simulink library "tqd"  (R2021b)
settings: Solver=VariableStepAuto  StartTime=0.0  StopTime=10.0  RelTol=1e-3
undefined symbols (not defined in the file or in its folder): ATQD_APSDecReq_X_kph, ATQD_APSDecReq_Y_mps2, ATQD_APSDecReqCMD_X_kph, ATQD_APSDecReqTs_X_pct, ATQD_APSDecTimeGain_X_Deg, ATQD_APSDecTimeGain_Y_s, ATQD_APSReqLowSpd_X_Deg, ATQD_AutoHoldReleaseBPS_X_Deg, ATQD_AWDLoadTrqnsGain_X_kg, ATQD_AWDLoadTrqnsGain_Y_pct, ATQD_BOSEnBPSPosn_X_kph, ATQD_BOSMap_X_rpm, ATQD_BOSMap_Y_pct, ATQD_CreepBaseTqD_X_kph, ATQD_CreepBaseTqD_Y_Deg, ATQD_CreepBaseTqR_X_kph, ATQD_CreepBaseTqR_Y_Deg, ATQD_CreepBPSDisPosn_X_Deg, ATQD_CreepBPSDisPosnR_X_Deg, ATQD_CreepBPSEnPosn_X_Deg, ATQD_CreepBPSEnPosnR_X_Deg, ATQD_CreepDeltaTq_X_kph, ATQD_CreepIterm_X_kph, ATQD_CreepIterm_Y_kph, ATQD_CreepItermMaxLimit_X_pct, ATQD_CreepPreloadTime_X_kph, ATQD_CreepPreloadTq_X_kph, ATQD_CreepPreloadTq_Y_s, ATQD_CreepProtTq_X_Deg, ATQD_CreepPterm_X_kph, ATQD_CreepPterm_Y_kph, ATQD_ECOTqMapD_X_rpm, ATQD_ECOTqMapD_Y_pct, ATQD_EOPDTqMapDCon_X_rpm, ATQD_EOPDTqMapDCon_Y_Deg, ATQD_EstInitVehWeight_X_c, ATQD_LHMRollGenMapD_X_rpm, ATQD_LHMRollGenMapD_Y_rpm, ATQD_LHMTqMapD_X_rpm, ATQD_LHMTqMapD_Y_pct, ATQD_NL1TqMapD_X_rpm, ATQD_NL1TqMapD_Y_pct, ATQD_NOPDTqMapDCon_X_rpm, ATQD_NOPDTqMapDCon_Y_Deg, ATQD_NRMRrEDUSpRat_X_rpm, ATQD_NRMRrEDUSpRat_Y_Nm, ATQD_OPDHoldDownRelDelay_X_Deg, ATQD_OPDHoldEnSpd_X_Deg, ATQD_OPDHoldRelDetTime_X_Deg, ATQD_OPDHoldReleaseTq_X_Deg, ATQD_OrigPedTqLowLim_X_Deg, ATQD_OrigPedTqLowLim_Y_pct, ATQD_PedalMapClimbUpLim_X_rpm, ATQD_PedalMapClimbUpLim_Y_Deg, ATQD_PreLoadTq_X_s, ATQD_RollGenMapEL1_X_rpm, ATQD_RollGenMapEL1_Y_rpm, ATQD_SL1TqMapD_X_rpm, ATQD_SL1TqMapD_Y_pct, ATQD_SlideRegenTqGain_X_Gps ... (+491)
libraries: hcu_lib x83, simulink x73, tqr x1
(part 19 of 19)

== stateflow chart tqd/TQD/TorqueDemand/Signal_convert/SWC2_Subsystem/Speed Setting Mode/MSA Speed Setting ON/MSASetSpd_241018 ==
  state MeterSpd
    state OFF_Error_Disable
      en:
      VTQD_MSASetSpd_raw32 =  min(VTQD_MSAActiveMetSpdHi_raw32, VTQD_SpdLim4SetSpd_raw32);
      VTQD_MSASetSpd_raw32 = max(VTQD_MSAActiveMetSpdLo_raw32, VTQD_MSASetSpd_raw32);
      VTQD_MSASavedSetSpd_raw32 = VTQD_MSASetSpd_raw32;
      du:
      VTQD_MSASetSpd_raw32 =  min(VTQD_MSAActiveMetSpdHi_raw32, VTQD_SpdLim4SetSpd_raw32);
      VTQD_MSASetSpd_raw32 = max(VTQD_MSAActiveMetSpdLo_raw32, VTQD_MSASetSpd_raw32);
      VTQD_MSASavedSetSpd_raw32 = VTQD_MSASetSpd_raw32;
    state Terminal
      %Do Nothing
    state Standby
      en:
      VTQD_MSASetSpd_raw32 =  min(VTQD_MSAActiveMetSpdHi_raw32, VTQD_SpdLim4SetSpd_raw32);
      VTQD_MSASetSpd_raw32 = max(VTQD_MSAActiveMetSpdLo_raw32, VTQD_MSASetSpd_raw32);
      VTQD_MSASavedSetSpd_raw32 = VTQD_MSASetSpd_raw32;
      du:
      VTQD_MSASetSpd_raw32 =  min(VTQD_MSAActiveMetSpdHi_raw32, VTQD_SpdLim4SetSpd_raw32);
      VTQD_MSASetSpd_raw32 = max(VTQD_MSAActiveMetSpdLo_raw32, VTQD_MSASetSpd_raw32);
      VTQD_MSASavedSetSpd_raw32 = VTQD_MSASetSpd_raw32;
    state Active_Override
      (default) -> (junction 749) : {VTQD_MSASetSpd_raw32 = VTQD_MSASavedSetSpd_raw32;}
      MeterSpd.Active_Override -> (junction 830) [order 1]
      (junction 830) -> (junction 834) [order 1] : [VTQD_DistanceUnit_flg == VINP_Distanceunit_flg || VTQD_MSASavedSetSpd_raw32 <= ONE_FLOAT]
      (junction 834) -> (junction 749) : {VTQD_MSASetSpd_raw32 = min(VTQD_MSAActiveMetSpdHi_raw32, VTQD_MSASavedSetSpd_raw32);
          |  VTQD_MSASavedSetSpd_raw32 = VTQD_MSASetSpd_raw32;}
      (junction 749) -> (junction 751) [order 1] : [VVMC_MSACrlSta_enum == ENUM_ADASMSASTA_ACTIVE]
      (junction 751) -> (junction 757) [order 1] : [VTQD_Set2MeterSpd_flg ||...
          |  VTQD_SetRoadSpdLim_flg]
      (junction 757) -> (junction 1111) [order 1] : [VTQD_Set2MeterSpd_flg]
      (junction 830) -> (junction 832) [order 2]
      (junction 837) -> (junction 834)
      (junction 749) -> (junction 798) [order 2]
      (junction 751) -> (junction 762) [order 2]
      (junction 757) -> (junction 759) [order 2] : {VTQD_MSASetSpd_raw32 =  min(VTQD_MSAActiveMetSpdHi_raw32, VTQD_SpdLim4SetSpd_raw32);
          |  VTQD_MSASetSpd_raw32 = max(VTQD_MSAActiveMetSpdLo_raw32, VTQD_MSASetSpd_raw32);
          |  VTQD_MSASavedSetSpd_raw32 = VTQD_MSASetSpd_raw32;
          |  VTQD_DistanceUnit_flg = VINP_Distanceunit_flg;}
      (junction 1111) -> (junction 1112) : {VTQD_MSASetSpd_raw32 =  min(VTQD_MSAActiveMetSpdHi_raw32, VVMC_MeterIndSpeed_raw32);
          |  VTQD_MSASetSpd_raw32 = max(VTQD_MSAActiveMetSpdLo_raw32, VTQD_MSASetSpd_raw32);
          |  VTQD_MSASavedSetSpd_raw32 = VTQD_MSASetSpd_raw32;
          |  VTQD_DistanceUnit_flg = VINP_Distanceunit_flg;}
      (junction 832) -> (junction 819) [order 1] : [VINP_Distanceunit_flg]
      (junction 832) -> (junction 833) [order 2] : {VTQD_MSASavedSetSpd_raw32 = (VTQD_MSASavedSetSpd_raw32 * MPH2KPH)}
      (junction 819) -> (junction 827) : {VTQD_MSASavedSetSpd_raw32 = (VTQD_MSASavedSetSpd_raw32 * KPH2MPH)}
      (junction 762) -> (junction 766) [order 1] : [(VTQD_SWC2ScrollUpSta_enum == ENUM_SWCBOTTONPRESS_SHORTPRESS ||...
          |   VTQD_SWC2ScrollDownSta_enum == ENUM_SWCBOTTONPRESS_SHORTPRESS)]
      (junction 766) -> (junction 771) [order 1] : [VTQD_SWC2ScrollUpSta_enum == ENUM_SWCBOTTONPRESS_SHORTPRESS]
      (junction 762) -> (junction 792) [order 2]
      (junction 766) -> (junction 779) [order 2] : {VTQD_MSASetSpd_raw32 =  min(VTQD_MSAActiveMetSpdHi_raw32, VTQD_MSASavedSetSpd_raw32 - ONE_FLOAT);
          |  VTQD_MSASetSpd_raw32 = max(VTQD_MSAActiveMetSpdLo_raw32, VTQD_MSASetSpd_raw32);
          |  VTQD_MSASavedSetSpd_raw32 = VTQD_MSASetSpd_raw32;
          |  VTQD_DistanceUnit_flg = VINP_Distanceunit_flg;}
      (junction 771) -> (junction 774) : {VTQD_MSASetSpd_raw32 =  min(VTQD_MSAActiveMetSpdHi_raw32, VTQD_MSASavedSetSpd_raw32 + ONE_FLOAT);
          |  VTQD_MSASetSpd_raw32 = max(VTQD_MSAActiveMetSpdLo_raw32, VTQD_MSASetSpd_raw32);
          |  VTQD_MSASavedSetSpd_raw32 = VTQD_MSASetSpd_raw32;
          |  VTQD_DistanceUnit_flg = VINP_Distanceunit_flg;}
      (junction 827) -> (junction 816) [order 1] : [VTQD_MSASavedSetSpd_raw32 < KTQD_MSAActiveMetSpdLoMPH_mph]
      (junction 833) -> (junction 817) [order 1] : [VTQD_MSASavedSetSpd_raw32 < KTQD_MSAActiveMetSpdLo_kph]
      (junction 816) -> (junction 820) : {VTQD_MSASavedSetSpd_raw32 = KTQD_MSAActiveMetSpdLoMPH_mph}
      (junction 833) -> (junction 828) [order 2]
      (junction 817) -> (junction 815) : {VTQD_MSASavedSetSpd_raw32 = KTQD_MSAActiveMetSpdLo_kph}
      (junction 827) -> (junction 818) [order 2]
      (junction 820) -> (junction 818)
      (junction 815) -> (junction 828)
      (junction 818) -> (junction 826)
      (junction 828) -> (junction 821)
      (junction 821) -> (junction 829) [order 1] : [VTQD_MSASavedSetSpd_raw32 > KTQD_MSAActiveMetSpdHi_kph]
      (junction 826) -> (junction 822) [order 1] : [VTQD_MSASavedSetSpd_raw32 > KTQD_MSAActiveMetSpdHiMPH_mph]
      (junction 821) -> (junction 823) [order 2]
      (junction 829) -> (junction 831) : {VTQD_MSASavedSetSpd_raw32 = KTQD_MSAActiveMetSpdHi_kph}
      (junction 826) -> (junction 835) [order 2]
      (junction 822) -> (junction 824) : {VTQD_MSASavedSetSpd_raw32 = KTQD_MSAActiveMetSpdHiMPH_mph}
      (junction 792) -> (junction 785) [order 1] : [(VTQD_SWC2ScrollUpSta_enum == ENUM_SWCBOTTONPRESS_LONGPRESS ||...
          |   VTQD_SWC2ScrollDownSta_enum == ENUM_SWCBOTTONPRESS_LONGPRESS)]
      (junction 785) -> (junction 790) [order 1] : [VTQD_SWC2ScrollUpSta_enum == ENUM_SWCBOTTONPRESS_LONGPRESS]
      (junction 831) -> (junction 823)
      (junction 824) -> (junction 835)
      (junction 785) -> (junction 793) [order 2] : {VTQD_MSASetSpd_raw32 = max(VTQD_MSAActiveMetSpdLo_raw32, ceil(VTQD_MSASavedSetSpd_raw32 / VTQD_SetSpdDeltaLong_raw32 - ONE_FLOAT) * VTQD_SetSpdDeltaLong_raw32);
          |  VTQD_MSASetSpd_raw32 = min (VTQD_MSAActiveMetSpdHi_raw32, VTQD_MSASetSpd_raw32);
          |  VTQD_MSASavedSetSpd_raw32 = VTQD_MSASetSpd_raw32;
          |  VTQD_DistanceUnit_flg = VINP_Distanceunit_flg;}
      (junction 792) -> (junction 809) [order 2] : {VTQD_MSASetSpd_raw32 = min(VTQD_MSAActiveMetSpdHi_raw32, ...
          |  VTQD_MSASavedSetSpd_raw32);
          |  VTQD_MSASetSpd_raw32 = max(VTQD_MSAActiveMetSpdLo_raw32, ...
          |  VTQD_MSASetSpd_raw32);
          |  VTQD_MSASavedSetSpd_raw32 = VTQD_MSASetSpd_raw32;
          |  VTQD_DistanceUnit_flg = VINP_Distanceunit_flg;}
          | %add20241113
      (junction 790) -> (junction 783) : {VTQD_MSASetSpd_raw32 = min(VTQD_MSAActiveMetSpdHi_raw32, floor(VTQD_MSASavedSetSpd_raw32 / VTQD_SetSpdDeltaLong_raw32 + ONE_FLOAT) * VTQD_SetSpdDeltaLong_raw32);
          |  VTQD_MSASetSpd_raw32 = max (VTQD_MSAActiveMetSpdLo_raw32, VTQD_MSASetSpd_raw32);
          |  VTQD_MSASavedSetSpd_raw32 = VTQD_MSASetSpd_raw32;
          |  VTQD_DistanceUnit_flg = VINP_Distanceunit_flg;}
      (junction 823) -> (junction 825)
      (junction 835) -> (junction 836)
      (junction 825) -> (junction 836)
      (junction 836) -> (junction 837)
      (junction 798) -> (junction 806) [order 1] : [VVMC_MSACrlSta_enum == ENUM_ADASMSASTA_UNLIMIT]
      (junction 806) -> (junction 804) [order 1] : [KTQD_ACCOVRDSpdAdj_flg &&...
          | (VTQD_Set2MeterSpd_flg ||...
          |  VTQD_SetRoadSpdLim_flg)]
      (junction 804) -> (junction 1115) [order 1] : [VTQD_Set2MeterSpd_flg]
      (junction 804) -> (junction 803) [order 2] : {VTQD_MSASetSpd_raw32 =  min(VTQD_MSAActiveMetSpdHi_raw32, VTQD_SpdLim4SetSpd_raw32);
          |  VTQD_MSASetSpd_raw32 = max(VTQD_MSAActiveMetSpdLo_raw32, VTQD_MSASetSpd_raw32);
          |  VTQD_MSASavedSetSpd_raw32 = VTQD_MSASetSpd_raw32;
          |  VTQD_DistanceUnit_flg = VINP_Distanceunit_flg;}
      (junction 1115) -> (junction 1116) : {VTQD_MSASetSpd_raw32 =  min(VTQD_MSAActiveMetSpdHi_raw32, VVMC_MeterIndSpeed_raw32);
          |  VTQD_MSASetSpd_raw32 = max(VTQD_MSAActiveMetSpdLo_raw32, VTQD_MSASetSpd_raw32);
          |  VTQD_MSASavedSetSpd_raw32 = VTQD_MSASetSpd_raw32;
          |  VTQD_DistanceUnit_flg = VINP_Distanceunit_flg;}
      (junction 798) -> (junction 807) [order 2] : {VTQD_MSASetSpd_raw32 = min(VTQD_MSAActiveMetSpdHi_raw32, ...
          |  VTQD_MSASavedSetSpd_raw32);
          |  VTQD_MSASetSpd_raw32 = max(VTQD_MSAActiveMetSpdLo_raw32, ...
          |  VTQD_MSASetSpd_raw32);
          |  VTQD_MSASavedSetSpd_raw32 = VTQD_MSASetSpd_raw32;
          |  VTQD_DistanceUnit_flg = VINP_Distanceunit_flg;}
          | %add20241113
      (junction 806) -> (junction 811) [order 2] : {VTQD_MSASetSpd_raw32 = min(VTQD_MSAActiveMetSpdHi_raw32, ...
          |  VTQD_MSASavedSetSpd_raw32);
          |  VTQD_MSASetSpd_raw32 = max(VTQD_MSAActiveMetSpdLo_raw32, ...
          |  VTQD_MSASetSpd_raw32);
          |  VTQD_MSASavedSetSpd_raw32 = VTQD_MSASetSpd_raw32;
          |  VTQD_DistanceUnit_flg = VINP_Distanceunit_flg;}
          | %add20241113
    (default) -> MeterSpd.OFF_Error_Disable [order 3]
    MeterSpd.Terminal -> MeterSpd.OFF_Error_Disable [order 2] : [VVMC_MSACrlSta_enum ~= ENUM_ADASMSASTA_ACTIVE &&...
        |  VVMC_MSACrlSta_enum ~= ENUM_ADASMSASTA_UNLIMIT]
    MeterSpd.OFF_Error_Disable -> MeterSpd.Terminal [order 2] : [VVMC_MSACrlSta_enum == ENUM_ADASMSASTA_ACTIVE ||...
        |  VVMC_MSACrlSta_enum == ENUM_ADASMSASTA_UNLIMIT]
    MeterSpd.Terminal -> MeterSpd.Active_Override [order 1] : [VVMC_MSACrlSta_enum == ENUM_ADASMSASTA_ACTIVE ||...
        |  VVMC_MSACrlSta_enum == ENUM_ADASMSASTA_UNLIMIT]
    MeterSpd.Active_Override -> MeterSpd.Terminal [order 2] : [VVMC_MSACrlSta_enum ~= ENUM_ADASMSASTA_ACTIVE &&...
        |  VVMC_MSACrlSta_enum ~= ENUM_ADASMSASTA_UNLIMIT]
    MeterSpd.OFF_Error_Disable -> MeterSpd.Standby [order 1] : [VVMC_MSACrlSta_enum == ENUM_ADASMSASTA_STANDBY]
    MeterSpd.Standby -> MeterSpd.OFF_Error_Disable [order 2] : [VVMC_MSACrlSta_enum ~= ENUM_ADASMSASTA_STANDBY]
    MeterSpd.Active_Override -> MeterSpd.Standby [order 1] : [VVMC_MSACrlSta_enum == ENUM_ADASMSASTA_STANDBY]
    MeterSpd.Standby -> MeterSpd.Active_Override [order 1] : [VVMC_MSACrlSta_enum == ENUM_ADASMSASTA_ACTIVE ||...
        |  VVMC_MSACrlSta_enum == ENUM_ADASMSASTA_UNLIMIT]
    (default) -> MeterSpd.Active_Override [order 2] : [VVMC_MSACrlSta_enum == ENUM_ADASMSASTA_ACTIVE ||...
        |  VVMC_MSACrlSta_enum == ENUM_ADASMSASTA_UNLIMIT]
    (default) -> MeterSpd.Standby [order 1] : [VVMC_MSACrlSta_enum == ENUM_ADASMSASTA_STANDBY]
  state RoadSpd
    state OFF_Error_Disable
      en:
      VTQD_MSASetSpd_raw32 =  min(VTQD_MSAActiveMetSpdHi_raw32, VTQD_SpdLim4SetSpd_raw32);
      VTQD_MSASetSpd_raw32 = max(VTQD_MSAActiveMetSpdLo_raw32, VTQD_MSASetSpd_raw32);
      VTQD_MSASavedSetSpd_raw32 = VTQD_MSASetSpd_raw32;
      du:
      VTQD_MSASetSpd_raw32 =  min(VTQD_MSAActiveMetSpdHi_raw32, VTQD_SpdLim4SetSpd_raw32);
      VTQD_MSASetSpd_raw32 = max(VTQD_MSAActiveMetSpdLo_raw32, VTQD_MSASetSpd_raw32);
      VTQD_MSASavedSetSpd_raw32 = VTQD_MSASetSpd_raw32;
    state Terminal
      %Do Nothing
    state Standby
      (default) -> (junction 987) : {VTQD_StandbyDisRoadSpd_flg = FALSE;}
      RoadSpd.Standby -> (junction 1029) [order 1]
      (junction 1029) -> (junction 1030) [order 1] : [VTQD_DistanceUnit_flg == VINP_Distanceunit_flg || VTQD_MSASavedSetSpd_raw32 <= ONE_FLOAT]
      (junction 1030) -> (junction 987) : {VTQD_MSASetSpd_raw32 = min(VTQD_MSAActiveMetSpdHi_raw32, VTQD_MSASavedSetSpd_raw32);
          |  VTQD_MSASavedSetSpd_raw32 = VTQD_MSASetSpd_raw32;}
      (junction 987) -> (junction 1102) [order 1] : [VTQD_RoadSpdActive2Standby_flg &&...
          | (VTQD_StandbyDisRoadSpd_flg || !VTQD_ADASSLIFSpdLimDet_flg)]
      (junction 1029) -> (junction 1031) [order 2]
      (junction 1048) -> (junction 1030)
      (junction 987) -> (junction 1104) [order 2]
      (junction 1102) -> (junction 999)
      (junction 1031) -> (junction 1032) [order 1] : [VINP_Distanceunit_flg]
      (junction 1031) -> (junction 1034) [order 2] : {VTQD_MSASavedSetSpd_raw32 = (VTQD_MSASavedSetSpd_raw32 * MPH2KPH)}
      (junction 1032) -> (junction 1028) : {VTQD_MSASavedSetSpd_raw32 = (VTQD_MSASavedSetSpd_raw32 * KPH2MPH)}
      (junction 1104) -> (junction 999) [order 1] : [VTQD_SWC2ScrollUpSta_enum ~= ENUM_SWCBOTTONPRESS_NOPRESS ||...
          |  VTQD_SWC2ScrollDownSta_enum ~= ENUM_SWCBOTTONPRESS_NOPRESS ||...
          |  VTQD_StandbyDisRoadSpd_flg]
      (junction 999) -> (junction 1000) [order 1] : [VTQD_SWC2ScrollUpSta_enum == ENUM_SWCBOTTONPRESS_SHORTPRESS ||...
          |  VTQD_SWC2ScrollDownSta_enum == ENUM_SWCBOTTONPRESS_SHORTPRESS]
      (junction 1000) -> (junction 1001) [order 1] : [VTQD_SWC2ScrollUpSta_enum == ENUM_SWCBOTTONPRESS_SHORTPRESS]
      (junction 1104) -> (junction 991) [order 2] : {VTQD_MSASetSpd_raw32 =  min(VTQD_MSAActiveMetSpdHi_raw32, VTQD_SpdLim4SetSpd_raw32);
          |  VTQD_MSASetSpd_raw32 = max(VTQD_MSAActiveMetSpdLo_raw32, VTQD_MSASetSpd_raw32);
          |  VTQD_MSASavedSetSpd_raw32 = VTQD_MSASetSpd_raw32;
          |  VTQD_DistanceUnit_flg = VINP_Distanceunit_flg;
          |  VTQD_RoadSpdActive2Standby_flg = FALSE;}
      (junction 999) -> (junction 1007) [order 2]
      (junction 1000) -> (junction 1005) [order 2] : {VTQD_MSASetSpd_raw32 =  min(VTQD_MSAActiveMetSpdHi_raw32, VTQD_MSASavedSetSpd_raw32 - ONE_FLOAT);
          |  VTQD_MSASetSpd_raw32 = max(VTQD_MSAActiveMetSpdLo_raw32, VTQD_MSASetSpd_raw32);
          |  VTQD_MSASavedSetSpd_raw32 = VTQD_MSASetSpd_raw32;
          |  VTQD_DistanceUnit_flg = VINP_Distanceunit_flg;
          |  VTQD_StandbyDisRoadSpd_flg = TRUE;}
      (junction 1001) -> (junction 1006) : {VTQD_MSASetSpd_raw32 =  min(VTQD_MSAActiveMetSpdHi_raw32, VTQD_MSASavedSetSpd_raw32 + ONE_FLOAT);
          |  VTQD_MSASetSpd_raw32 = max(VTQD_MSAActiveMetSpdLo_raw32, VTQD_MSASetSpd_raw32);
          |  VTQD_MSASavedSetSpd_raw32 = VTQD_MSASetSpd_raw32;
          |  VTQD_DistanceUnit_flg = VINP_Distanceunit_flg;
          |  VTQD_StandbyDisRoadSpd_flg = TRUE;}
      (junction 1028) -> (junction 1033) [order 1] : [VTQD_MSASavedSetSpd_raw32 < KTQD_MSAActiveMetSpdLoMPH_mph]
      (junction 1034) -> (junction 1035) [order 1] : [VTQD_MSASavedSetSpd_raw32 < KTQD_MSAActiveMetSpdLo_kph]
      (junction 1033) -> (junction 1043) : {VTQD_MSASavedSetSpd_raw32 = KTQD_MSAActiveMetSpdLoMPH_mph}
      (junction 1034) -> (junction 1038) [order 2]
      (junction 1035) -> (junction 1039) : {VTQD_MSASavedSetSpd_raw32 = KTQD_MSAActiveMetSpdLo_kph}
      (junction 1028) -> (junction 1045) [order 2]
      (junction 1043) -> (junction 1045)
      (junction 1039) -> (junction 1038)
      (junction 1045) -> (junction 1042)
      (junction 1038) -> (junction 1040)
      (junction 1040) -> (junction 1041) [order 1] : [VTQD_MSASavedSetSpd_raw32 > KTQD_MSAActiveMetSpdHi_kph]
      (junction 1042) -> (junction 1044) [order 1] : [VTQD_MSASavedSetSpd_raw32 > KTQD_MSAActiveMetSpdHiMPH_mph]
      (junction 1040) -> (junction 1053) [order 2]
      (junction 1041) -> (junction 1049) : {VTQD_MSASavedSetSpd_raw32 = KTQD_MSAActiveMetSpdHi_kph}
      (junction 1042) -> (junction 1054) [order 2]
      (junction 1044) -> (junction 1047) : {VTQD_MSASavedSetSpd_raw32 = KTQD_MSAActiveMetSpdHiMPH_mph}
      (junction 1007) -> (junction 1011) [order 1] : [VTQD_SWC2ScrollUpSta_enum == ENUM_SWCBOTTONPRESS_LONGPRESS ||...
          |  VTQD_SWC2ScrollDownSta_enum == ENUM_SWCBOTTONPRESS_LONGPRESS]
      (junction 1011) -> (junction 1009) [order 1] : [VTQD_SWC2ScrollUpSta_enum == ENUM_SWCBOTTONPRESS_LONGPRESS]
      (junction 1007) -> (junction 1012) [order 2]
      (junction 1011) -> (junction 1010) [order 2] : {VTQD_MSASetSpd_raw32 = max(VTQD_MSAActiveMetSpdLo_raw32, ceil(VTQD_MSASavedSetSpd_raw32 / VTQD_SetSpdDeltaLong_raw32 - ONE_FLOAT) * VTQD_SetSpdDeltaLong_raw32);
          |  VTQD_MSASetSpd_raw32 = min (VTQD_MSAActiveMetSpdHi_raw32, VTQD_MSASetSpd_raw32);
          |  VTQD_MSASavedSetSpd_raw32 = VTQD_MSASetSpd_raw32;
          |  VTQD_DistanceUnit_flg = VINP_Distanceunit_flg;
          |  VTQD_StandbyDisRoadSpd_flg = TRUE;}
      (junction 1009) -> (junction 1008) : {VTQD_MSASetSpd_raw32 = min(VTQD_MSAActiveMetSpdHi_raw32, floor(VTQD_MSASavedSetSpd_raw32 / VTQD_SetSpdDeltaLong_raw32 + ONE_FLOAT) * VTQD_SetSpdDeltaLong_raw32);
          |  VTQD_MSASetSpd_raw32 = max (VTQD_MSAActiveMetSpdLo_raw32, VTQD_MSASetSpd_raw32);
          |  VTQD_MSASavedSetSpd_raw32 = VTQD_MSASetSpd_raw32;
          |  VTQD_DistanceUnit_flg = VINP_Distanceunit_flg;
          |  VTQD_StandbyDisRoadSpd_flg = TRUE;}
      (junction 1049) -> (junction 1053)
      (junction 1047) -> (junction 1054)
      (junction 1053) -> (junction 1046)
      (junction 1054) -> (junction 1050)
      (junction 1046) -> (junction 1050)
      (junction 1050) -> (junction 1048)
      (junction 1012) -> (junction 1023) [order 1] : [VTQD_LScrollPressShort_flg &&...
          |  VTQD_ADASSLIFSpdLimDet_flg]
      (junction 1023) -> (junction 1026) : {VTQD_MSASetSpd_raw32 =  min(VTQD_MSAActiveMetSpdHi_raw32, VTQD_SpdLim4SetSpd_raw32);
          |  VTQD_MSASetSpd_raw32 = max(VTQD_MSAActiveMetSpdLo_raw32, VTQD_MSASetSpd_raw32);
          |  VTQD_MSASavedSetSpd_raw32 = VTQD_MSASetSpd_raw32;
          |  VTQD_DistanceUnit_flg = VINP_Distanceunit_flg;
          |  VTQD_StandbyDisRoadSpd_flg = FALSE;
          |  VTQD_RoadSpdActive2Standby_flg = FALSE;}
      (junction 1012) -> (junction 1022) [order 2] : {VTQD_MSASetSpd_raw32 =  VTQD_MSASavedSetSpd_raw32;
          |  VTQD_MSASavedSetSpd_raw32 = VTQD_MSASetSpd_raw32;
          |  VTQD_DistanceUnit_flg = VINP_Distanceunit_flg;}
    state Active_Override
      (default) -> (junction 883) : {VTQD_MSASetSpd_raw32 = VTQD_MSASavedSetSpd_raw32;}
      RoadSpd.Active_Override -> (junction 881) [order 1]
      (junction 881) -> (junction 882) [order 1] : [VTQD_DistanceUnit_flg == VINP_Distanceunit_flg || VTQD_MSASavedSetSpd_raw32 <= ONE_FLOAT]
      (junction 882) -> (junction 883) : {VTQD_MSASetSpd_raw32 = min(VTQD_MSAActiveMetSpdHi_raw32, VTQD_MSASavedSetSpd_raw32);
          |  VTQD_MSASavedSetSpd_raw32 = VTQD_MSASetSpd_raw32;}
      (junction 883) -> (junction 884) [order 1] : [VVMC_MSACrlSta_enum == ENUM_ADASMSASTA_ACTIVE]
      (junction 884) -> (junction 885) [order 1] : [VTQD_Set2MeterSpd_flg ||...
          |  VTQD_SetRoadSpdLim_flg]
      (junction 885) -> (junction 1120) [order 1] : [VTQD_Set2MeterSpd_flg]
      (junction 881) -> (junction 886) [order 2]
      (junction 915) -> (junction 882)
      (junction 883) -> (junction 919) [order 2]
      (junction 884) -> (junction 889) [order 2]
      (junction 885) -> (junction 888) [order 2] : {VTQD_MSASetSpd_raw32 =  min(VTQD_MSAActiveMetSpdHi_raw32, VTQD_SpdLim4SetSpd_raw32);
          |  VTQD_MSASetSpd_raw32 = max(VTQD_MSAActiveMetSpdLo_raw32, VTQD_MSASetSpd_raw32);
          |  VTQD_MSASavedSetSpd_raw32 = VTQD_MSASetSpd_raw32;
          |  VTQD_DistanceUnit_flg = VINP_Distanceunit_flg;}
      (junction 1120) -> (junction 1119) : {VTQD_MSASetSpd_raw32 =  min(VTQD_MSAActiveMetSpdHi_raw32, VVMC_MeterIndSpeed_raw32);
          |  VTQD_MSASetSpd_raw32 = max(VTQD_MSAActiveMetSpdLo_raw32, VTQD_MSASetSpd_raw32);
          |  VTQD_MSASavedSetSpd_raw32 = VTQD_MSASetSpd_raw32;
          |  VTQD_DistanceUnit_flg = VINP_Distanceunit_flg;}
      (junction 886) -> (junction 887) [order 1] : [VINP_Distanceunit_flg]
      (junction 886) -> (junction 893) [order 2] : {VTQD_MSASavedSetSpd_raw32 = (VTQD_MSASavedSetSpd_raw32 * MPH2KPH)}
      (junction 887) -> (junction 895) : {VTQD_MSASavedSetSpd_raw32 = (VTQD_MSASavedSetSpd_raw32 * KPH2MPH)}
      (junction 889) -> (junction 890) [order 1] : [(VTQD_SWC2ScrollUpSta_enum == ENUM_SWCBOTTONPRESS_SHORTPRESS ||...
          |   VTQD_SWC2ScrollDownSta_enum == ENUM_SWCBOTTONPRESS_SHORTPRESS)]
      (junction 890) -> (junction 891) [order 1] : [VTQD_SWC2ScrollUpSta_enum == ENUM_SWCBOTTONPRESS_SHORTPRESS]
      (junction 889) -> (junction 906) [order 2]
      (junction 890) -> (junction 904) [order 2] : {VTQD_MSASetSpd_raw32 =  min(VTQD_MSAActiveMetSpdHi_raw32, VTQD_MSASavedSetSpd_raw32 - ONE_FLOAT);
          |  VTQD_MSASetSpd_raw32 = max(VTQD_MSAActiveMetSpdLo_raw32, VTQD_MSASetSpd_raw32);
          |  VTQD_MSASavedSetSpd_raw32 = VTQD_MSASetSpd_raw32;
          |  VTQD_DistanceUnit_flg = VINP_Distanceunit_flg;}
      (junction 891) -> (junction 905) : {VTQD_MSASetSpd_raw32 =  min(VTQD_MSAActiveMetSpdHi_raw32, VTQD_MSASavedSetSpd_raw32 + ONE_FLOAT);
          |  VTQD_MSASetSpd_raw32 = max(VTQD_MSAActiveMetSpdLo_raw32, VTQD_MSASetSpd_raw32);
          |  VTQD_MSASavedSetSpd_raw32 = VTQD_MSASetSpd_raw32;
          |  VTQD_DistanceUnit_flg = VINP_Distanceunit_flg;}
      (junction 895) -> (junction 892) [order 1] : [VTQD_MSASavedSetSpd_raw32 < KTQD_MSAActiveMetSpdLoMPH_mph]
      (junction 893) -> (junction 894) [order 1] : [VTQD_MSASavedSetSpd_raw32 < KTQD_MSAActiveMetSpdLo_kph]
      (junction 892) -> (junction 897) : {VTQD_MSASavedSetSpd_raw32 = KTQD_MSAActiveMetSpdLoMPH_mph}
      (junction 893) -> (junction 898) [order 2]
      (junction 894) -> (junction 899) : {VTQD_MSASavedSetSpd_raw32 = KTQD_MSAActiveMetSpdLo_kph}
      (junction 895) -> (junction 896) [order 2]
      (junction 897) -> (junction 896)
      (junction 899) -> (junction 898)
      (junction 896) -> (junction 902)
      (junction 898) -> (junction 900)
      (junction 900) -> (junction 901) [order 1] : [VTQD_MSASavedSetSpd_raw32 > KTQD_MSAActiveMetSpdHi_kph]
      (junction 902) -> (junction 903) [order 1] : [VTQD_MSASavedSetSpd_raw32 > KTQD_MSAActiveMetSpdHiMPH_mph]
      (junction 900) -> (junction 909) [order 2]
      (junction 901) -> (junction 910) : {VTQD_MSASavedSetSpd_raw32 = KTQD_MSAActiveMetSpdHi_kph}
      (junction 902) -> (junction 911) [order 2]
      (junction 903) -> (junction 912) : {VTQD_MSASavedSetSpd_raw32 = KTQD_MSAActiveMetSpdHiMPH_mph}
      (junction 906) -> (junction 907) [order 1] : [(VTQD_SWC2ScrollUpSta_enum == ENUM_SWCBOTTONPRESS_LONGPRESS ||...
          |   VTQD_SWC2ScrollDownSta_enum == ENUM_SWCBOTTONPRESS_LONGPRESS)]
      (junction 907) -> (junction 908) [order 1] : [VTQD_SWC2ScrollUpSta_enum == ENUM_SWCBOTTONPRESS_LONGPRESS]
      (junction 910) -> (junction 909)
      (junction 912) -> (junction 911)
      (junction 906) -> (junction 916) [order 2] : {VTQD_MSASetSpd_raw32 = VTQD_MSASavedSetSpd_raw32;
          |  VTQD_MSASavedSetSpd_raw32 = VTQD_MSASetSpd_raw32;
          |  VTQD_DistanceUnit_flg = VINP_Distanceunit_flg;}
      (junction 907) -> (junction 917) [order 2] : {VTQD_MSASetSpd_raw32 = max(VTQD_MSAActiveMetSpdLo_raw32, ceil(VTQD_MSASavedSetSpd_raw32 / VTQD_SetSpdDeltaLong_raw32 - ONE_FLOAT) * VTQD_SetSpdDeltaLong_raw32);
          |  VTQD_MSASetSpd_raw32 = min (VTQD_MSAActiveMetSpdHi_raw32, VTQD_MSASetSpd_raw32);
          |  VTQD_MSASavedSetSpd_raw32 = VTQD_MSASetSpd_raw32;
          |  VTQD_DistanceUnit_flg = VINP_Distanceunit_flg;}
      (junction 908) -> (junction 918) : {VTQD_MSASetSpd_raw32 = min(VTQD_MSAActiveMetSpdHi_raw32, floor(VTQD_MSASavedSetSpd_raw32 / VTQD_SetSpdDeltaLong_raw32 + ONE_FLOAT) * VTQD_SetSpdDeltaLong_raw32);
          |  VTQD_MSASetSpd_raw32 = max (VTQD_MSAActiveMetSpdLo_raw32, VTQD_MSASetSpd_raw32);
          |  VTQD_MSASavedSetSpd_raw32 = VTQD_MSASetSpd_raw32;
          |  VTQD_DistanceUnit_flg = VINP_Distanceunit_flg;}
      (junction 909) -> (junction 913)
      (junction 911) -> (junction 914)
      (junction 913) -> (junction 914)
      (junction 914) -> (junction 915)
      (junction 919) -> (junction 920) [order 1] : [VVMC_MSACrlSta_enum == ENUM_ADASMSASTA_UNLIMIT]
      (junction 920) -> (junction 921) [order 1] : [KTQD_ACCOVRDSpdAdj_flg &&...
          | (VTQD_Set2MeterSpd_flg ||...
          |  VTQD_SetRoadSpdLim_flg)]
      (junction 921) -> (junction 1124) [order 1] : [VTQD_Set2MeterSpd_flg]
      (junction 919) -> (junction 924) [order 2] : {VTQD_MSASetSpd_raw32 = VTQD_MSASavedSetSpd_raw32;
          |  VTQD_MSASavedSetSpd_raw32 = VTQD_MSASetSpd_raw32;
          |  VTQD_DistanceUnit_flg = VINP_Distanceunit_flg;}
      (junction 920) -> (junction 922) [order 2] : {VTQD_MSASetSpd_raw32 = VTQD_MSASavedSetSpd_raw32;
          |  VTQD_MSASavedSetSpd_raw32 = VTQD_MSASetSpd_raw32;
          |  VTQD_DistanceUnit_flg = VINP_Distanceunit_flg;}
      (junction 921) -> (junction 923) [order 2] : {VTQD_MSASetSpd_raw32 =  min(VTQD_MSAActiveMetSpdHi_raw32, VTQD_SpdLim4SetSpd_raw32);
          |  VTQD_MSASetSpd_raw32 = max(VTQD_MSAActiveMetSpdLo_raw32, VTQD_MSASetSpd_raw32);
          |  VTQD_MSASavedSetSpd_raw32 = VTQD_MSASetSpd_raw32;
          |  VTQD_DistanceUnit_flg = VINP_Distanceunit_flg;}
      (junction 1124) -> (junction 1123) : {VTQD_MSASetSpd_raw32 =  min(VTQD_MSAActiveMetSpdHi_raw32, VVMC_MeterIndSpeed_raw32);
          |  VTQD_MSASetSpd_raw32 = max(VTQD_MSAActiveMetSpdLo_raw32, VTQD_MSASetSpd_raw32);
          |  VTQD_MSASavedSetSpd_raw32 = VTQD_MSASetSpd_raw32;
          |  VTQD_DistanceUnit_flg = VINP_Distanceunit_flg;}
    (default) -> RoadSpd.OFF_Error_Disable [order 3]
    RoadSpd.Terminal -> RoadSpd.OFF_Error_Disable [order 2] : [VVMC_MSACrlSta_enum ~= ENUM_ADASMSASTA_ACTIVE &&...
        |  VVMC_MSACrlSta_enum ~= ENUM_ADASMSASTA_UNLIMIT]
    RoadSpd.OFF_Error_Disable -> RoadSpd.Terminal [order 2] : [VVMC_MSACrlSta_enum == ENUM_ADASMSASTA_ACTIVE ||...
        |  VVMC_MSACrlSta_enum == ENUM_ADASMSASTA_UNLIMIT]
        | {VTQD_RoadSpdActive2Standby_flg = FALSE;}
    RoadSpd.Terminal -> RoadSpd.Active_Override [order 1] : [VVMC_MSACrlSta_enum == ENUM_ADASMSASTA_ACTIVE ||...
        |  VVMC_MSACrlSta_enum == ENUM_ADASMSASTA_UNLIMIT]
    RoadSpd.Active_Override -> RoadSpd.Terminal [order 2] : [VVMC_MSACrlSta_enum ~= ENUM_ADASMSASTA_ACTIVE &&...
        |  VVMC_MSACrlSta_enum ~= ENUM_ADASMSASTA_UNLIMIT]
    RoadSpd.OFF_Error_Disable -> RoadSpd.Standby [order 1] : [VVMC_MSACrlSta_enum == ENUM_ADASMSASTA_STANDBY]
    RoadSpd.Standby -> RoadSpd.OFF_Error_Disable [order 2] : [VVMC_MSACrlSta_enum ~= ENUM_ADASMSASTA_STANDBY]
        | {VTQD_RoadSpdActive2Standby_flg = FALSE;}
    RoadSpd.Active_Override -> RoadSpd.Standby [order 1] : [VVMC_MSACrlSta_enum == ENUM_ADASMSASTA_STANDBY]
        | {VTQD_RoadSpdActive2Standby_flg = TRUE;}
    RoadSpd.Standby -> RoadSpd.Active_Override [order 1] : [VVMC_MSACrlSta_enum == ENUM_ADASMSASTA_ACTIVE ||...
        |  VVMC_MSACrlSta_enum == ENUM_ADASMSASTA_UNLIMIT]
        | {VTQD_RoadSpdActive2Standby_flg = FALSE;}
    (default) -> RoadSpd.Active_Override [order 2] : [VVMC_MSACrlSta_enum == ENUM_ADASMSASTA_ACTIVE ||...
        |  VVMC_MSACrlSta_enum == ENUM_ADASMSASTA_UNLIMIT]
    (default) -> RoadSpd.Standby [order 1] : [VVMC_MSACrlSta_enum == ENUM_ADASMSASTA_STANDBY]
  (default) -> MeterSpd : {VTQD_MSASavedSetSpd_raw32 = ZERO_FLOAT;
      |  VTQD_RoadSpdActive2Standby_flg = FALSE;
      |  VTQD_StandbyDisRoadSpd_flg = FALSE}
  RoadSpd -> MeterSpd : [!VINP_IVIACCAdaptiveSta_flg]
  MeterSpd -> RoadSpd : [VINP_IVIACCAdaptiveSta_flg]
  data: VVMC_MSACrlSta_enum input; ENUM_ADASMSASTA_STANDBY parameter; ENUM_ADASMSASTA_UNLIMIT parameter; ENUM_ADASMSASTA_ACTIVE parameter; ZERO_FLOAT parameter; VTQD_MSASetSpd_raw32 output single; VINP_IVIACCAdaptiveSta_flg input; VTQD_SpdLim4SetSpd_raw32 input; VTQD_MSAActiveMetSpdHi_raw32 input; VTQD_MSAActiveMetSpdLo_raw32 input; VTQD_Set2MeterSpd_flg input; VTQD_SWC2ScrollUpSta_enum input; VTQD_SWC2ScrollDownSta_enum input; ENUM_SWCBOTTONPRESS_SHORTPRESS parameter; ONE_FLOAT parameter; ENUM_SWCBOTTONPRESS_LONGPRESS parameter; VTQD_MSASavedSetSpd_raw32 local double; VTQD_SetSpdDeltaLong_raw32 input; VTQD_SetRoadSpdLim_flg input; KTQD_ACCOVRDSpdAdj_flg parameter; KPH2MPH parameter; VTQD_DistanceUnit_flg local boolean; MPH2KPH parameter; KTQD_MSAActiveMetSpdHiMPH_mph parameter; KTQD_MSAActiveMetSpdHi_kph parameter; KTQD_MSAActiveMetSpdLoMPH_mph parameter; KTQD_MSAActiveMetSpdLo_kph parameter; VTQD_RoadSpdActive2Standby_flg local boolean; VINP_Distanceunit_flg input; VTQD_ADASSLIFSpdLimDet_flg input; VTQD_StandbyDisRoadSpd_flg local boolean; VTQD_LScrollPressShort_flg input; FALSE parameter; TRUE parameter; ENUM_SWCBOTTONPRESS_NOPRESS parameter; VVMC_MeterIndSpeed_raw32 input

== stateflow chart tqd/TQD/TorqueDemand/Signal_convert/SWC2_Subsystem/Speed Setting Mode/MSA Speed Setting ON/Specific_STATE_ChangeToOFF ==
  state FLG_ON
    en:
    VTQD_ChangeToOFF_flg = TRUE;
  state Initialize
    en:
    VTQD_ChangeToOFF_flg = FALSE;
  state STAY
  (default) -> Initialize
  Initialize -> STAY : [VINP_MSACrlSta_enum == ENUM_ADASMSASTA_UNLIMIT ||...
      | VINP_MSACrlSta_enum == ENUM_ADASMSASTA_ACTIVE]
  STAY -> FLG_ON [order 1] : [VINP_MSACrlSta_enum == ENUM_ADASMSASTA_STANDBY]
  STAY -> Initialize [order 2] : [VINP_MSACrlSta_enum != ENUM_ADASMSASTA_STANDBY &&...
      | VINP_MSACrlSta_enum != ENUM_ADASMSASTA_ACTIVE&&...
      | VINP_MSACrlSta_enum != ENUM_ADASMSASTA_UNLIMIT]
  (junction 11) -> Initialize
  FLG_ON -> (junction 9)
  (junction 9) -> (junction 11) : [VINP_MSACrlSta_enum != ENUM_ADASMSASTA_STANDBY]
  data: VINP_MSACrlSta_enum input; VTQD_ChangeToOFF_flg output boolean; FALSE parameter; TRUE parameter; ENUM_ADASMSASTA_ACTIVE parameter; ENUM_ADASMSASTA_STANDBY parameter; ENUM_ADASMSASTA_UNLIMIT parameter
